simulink model "Untitled1"  (R2022a)
settings: Solver=VariableStepAuto  StartTime=0.0  StopTime=20  RelTol=1e-3
undefined symbols (not defined in the file or in its folder): X, Y, Z
libraries: sm_lib x10, nesl_utility x6
settings Model: SimulationMode=accelerator  Creator=alessiofranci  LastModifiedBy=alessiofranci

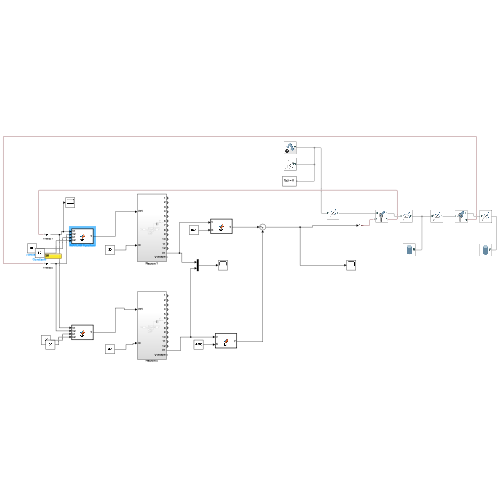
[thumbnail: Simulink's stored preview of the top-level diagram]
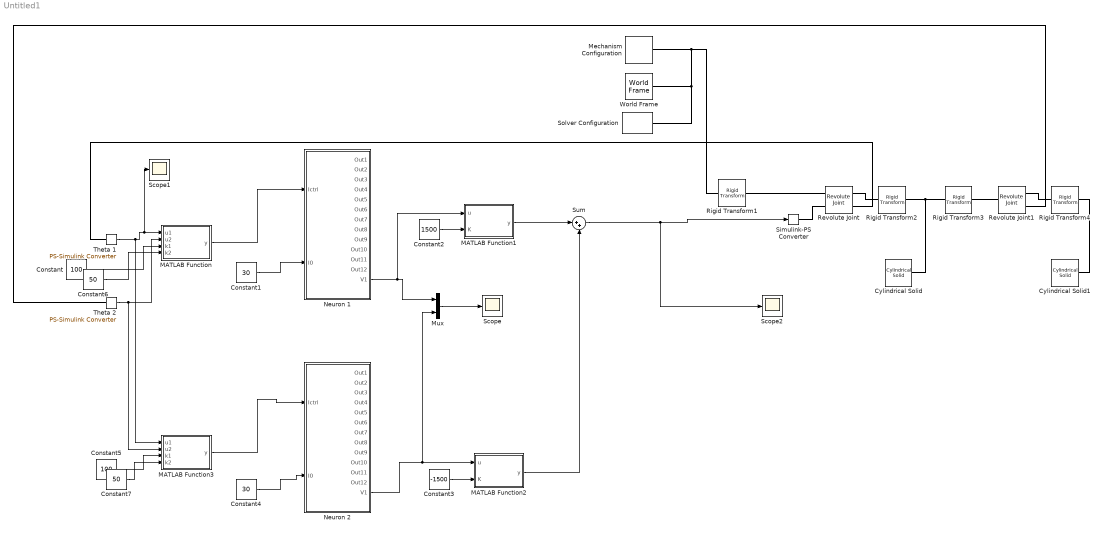
== system Untitled1 ==
  Constant : Constant  Value=100
  Constant1 : Constant  Value=30
  Constant2 : Constant  Value=1500
  Constant3 : Constant  Value=-1500
  Constant4 : Constant  Value=30
  Constant5 : Constant  Value=100
  Constant6 : Constant  Value=50
  Constant7 : Constant  Value=50
  Cylindrical Solid : sm_lib/Body Elements/Cylindrical Solid  GraphicAmbientColor=[0.15 0.15 0.15 1.0]  BasedOnType=Density  CenterOfMass=[0 0 0]  CenterOfMassUnits=m  GraphicDiffuseColor=[0.5 0.5 0.5]  CylinderLength=0.5  CylinderLengthUnits=m  CylinderRadius=0.05  CylinderRadiusUnits=m  Density=1000  DensityUnits=kg/m^3  DoExposeReferenceFrame=on  GraphicEmissiveColor=[0.0 0.0 0.0 1.0]  ExportEntireGeometry=off  SerializedFrames=<Frames/>  MarkerShape=Sphere  MarkerSize=10  GraphicType=FromGeometry  InertiaType=CalculateFromGeometry  Mass=1  MassUnits=kg  MomentsOfInertia=[1 1 1]  MomentsOfInertiaUnits=kg*m^2  GraphicOpacity=1.0  ProductsOfInertia=[0 0 0]  ProductsOfInertiaUnits=kg*m^2  GraphicShininess=75  GraphicSpecularColor=[0.5 0.5 0.5 1.0]  GraphicVisPropType=SimpleVisualProperties
  Cylindrical Solid1 : sm_lib/Body Elements/Cylindrical Solid  GraphicAmbientColor=[0.15 0.15 0.15 1.0]  BasedOnType=Density  CenterOfMass=[0 0 0]  CenterOfMassUnits=m  GraphicDiffuseColor=[0.5 0.5 0.5]  CylinderLength=0.5  CylinderLengthUnits=m  CylinderRadius=0.05  CylinderRadiusUnits=m  Density=1000  DensityUnits=kg/m^3  DoExposeReferenceFrame=on  GraphicEmissiveColor=[0.0 0.0 0.0 1.0]  ExportEntireGeometry=off  SerializedFrames=<Frames/>  MarkerShape=Sphere  MarkerSize=10  GraphicType=FromGeometry  InertiaType=CalculateFromGeometry  Mass=1  MassUnits=kg  MomentsOfInertia=[1 1 1]  MomentsOfInertiaUnits=kg*m^2  GraphicOpacity=1.0  ProductsOfInertia=[0 0 0]  ProductsOfInertiaUnits=kg*m^2  GraphicShininess=75  GraphicSpecularColor=[0.5 0.5 0.5 1.0]  GraphicVisPropType=SimpleVisualProperties
  MATLAB Function : MATLAB Function  TreatAsAtomicUnit=on
  MATLAB Function1 : MATLAB Function  TreatAsAtomicUnit=on
  MATLAB Function2 : MATLAB Function  TreatAsAtomicUnit=on
  MATLAB Function3 : MATLAB Function  TreatAsAtomicUnit=on
  Mechanism Configuration : sm_lib/Utilities/Mechanism Configuration  UniformGravity=Constant  GravityVector=[0 0 -9.80665]  GravityUnits=m/s^2  LinearizationDelta=0.001  JointModeTransitionNonlinearIterations=2
  Mux : Mux  Inputs=2
  Neuron 1 : Subsystem
  Neuron 2 : Subsystem
  Revolute Joint : sm_lib/Joints/Revolute Joint  JointMode=Normal  SenseConstraintForce=off  SenseConstraintForceX=off  SenseConstraintForceY=off  SenseConstraintForceZ=off  SenseConstraintTorque=off  SenseConstraintTorqueX=off  SenseConstraintTorqueY=off  SenseConstraintTorqueZ=off  SenseTotalForce=off  SenseTotalForceX=off  SenseTotalForceY=off  SenseTotalForceZ=off  SenseTotalTorque=off  SenseTotalTorqueX=off  SenseTotalTorqueY=off  SenseTotalTorqueZ=off  CompositeWrenchDir=FollowerOnBase  CompositeWrenchFrame=BaseFrame  EquilibriumPosition=0  EquilibriumPositionUnits=deg  SpringStiffness=0.0  SpringStiffnessUnits=N*m/deg  DampingCoefficient=0.0  DampingCoefficientUnits=N*m/(deg/s)  TorqueActuationMode=InputTorque  MotionActuationMode=ComputedMotion  SensePosition=on  SenseVelocity=off  SenseAcceleration=off  SenseTorqueForce=off  SenseLowerLimitTorqueForce=off  SenseUpperLimitTorqueForce=off  LowerLimitSpecify=off  LowerLimitBound=-90  LowerLimitBoundUnits=deg  LowerLimitStiffness=1e4  LowerLimitStiffnessUnits=N*m/deg  LowerLimitDamping=10  LowerLimitDampingUnits=N*m/(deg/s)  LowerLimitTransitionRegionWidth=0.1  LowerLimitTransitionRegionWidthUnits=deg  UpperLimitSpecify=off  UpperLimitBound=90  UpperLimitBoundUnits=deg  UpperLimitStiffness=1e4  UpperLimitStiffnessUnits=N*m/deg  UpperLimitDamping=10  UpperLimitDampingUnits=N*m/(deg/s)  UpperLimitTransitionRegionWidth=0.1  UpperLimitTransitionRegionWidthUnits=deg  PositionTargetSpecify=on  PositionTargetPriority=High  PositionTargetValue=20  PositionTargetValueUnits=deg  VelocityTargetSpecify=off  VelocityTargetPriority=High  VelocityTargetValue=0  VelocityTargetValueUnits=deg/s
  Revolute Joint1 : sm_lib/Joints/Revolute Joint  JointMode=Normal  SenseConstraintForce=off  SenseConstraintForceX=off  SenseConstraintForceY=off  SenseConstraintForceZ=off  SenseConstraintTorque=off  SenseConstraintTorqueX=off  SenseConstraintTorqueY=off  SenseConstraintTorqueZ=off  SenseTotalForce=off  SenseTotalForceX=off  SenseTotalForceY=off  SenseTotalForceZ=off  SenseTotalTorque=off  SenseTotalTorqueX=off  SenseTotalTorqueY=off  SenseTotalTorqueZ=off  CompositeWrenchDir=FollowerOnBase  CompositeWrenchFrame=BaseFrame  EquilibriumPosition=0  EquilibriumPositionUnits=deg  SpringStiffness=0.0  SpringStiffnessUnits=N*m/deg  DampingCoefficient=0.0  DampingCoefficientUnits=N*m/(deg/s)  TorqueActuationMode=NoTorque  MotionActuationMode=ComputedMotion  SensePosition=on  SenseVelocity=off  SenseAcceleration=off  SenseTorqueForce=off  SenseLowerLimitTorqueForce=off  SenseUpperLimitTorqueForce=off  LowerLimitSpecify=off  LowerLimitBound=-90  LowerLimitBoundUnits=deg  LowerLimitStiffness=1e4  LowerLimitStiffnessUnits=N*m/deg  LowerLimitDamping=10  LowerLimitDampingUnits=N*m/(deg/s)  LowerLimitTransitionRegionWidth=0.1  LowerLimitTransitionRegionWidthUnits=deg  UpperLimitSpecify=off  UpperLimitBound=90  UpperLimitBoundUnits=deg  UpperLimitStiffness=1e4  UpperLimitStiffnessUnits=N*m/deg  UpperLimitDamping=10  UpperLimitDampingUnits=N*m/(deg/s)  UpperLimitTransitionRegionWidth=0.1  UpperLimitTransitionRegionWidthUnits=deg  PositionTargetSpecify=on  PositionTargetPriority=High  PositionTargetValue=-20  PositionTargetValueUnits=deg  VelocityTargetSpecify=off  VelocityTargetPriority=High  VelocityTargetValue=0  VelocityTargetValueUnits=deg/s
  Rigid Transform1 : sm_lib/Frames and Transforms/Rigid Transform  TranslationMethod=None  TranslationStandardOffset=0.25  TranslationLengthUnit=m  TranslationStandardAxis=+X  TranslationCartesianOffset=[0 0 0]  TranslationROffset=0  TranslationROffsetUnits=m  TranslationZOffset=0  TranslationZOffsetUnits=m  TranslationThetaOffset=0  TranslationThetaOffsetUnits=deg  RotationMethod=RotationSequence  RotationAngleUnits=deg  RotationStandardAxis=+Y  RotationAngle=90  RotationArbitraryAxis=[0 0 1]  FollAlignAxisA=+X  BaseAlignAxisA=+Y  FollAlignAxisB=+Y  BaseAlignAxisB=+Z  RotationSequenceAxes=FollowerAxes  RotationSequence=XYX  RotationSequenceAngles=[0 90 90]  RotationSequenceAnglesUnits=deg  RotationMatrix=[1 0 0; 0 1 0; 0 0 1]
  Rigid Transform2 : sm_lib/Frames and Transforms/Rigid Transform  TranslationMethod=StandardAxis  TranslationStandardOffset=.25  TranslationLengthUnit=m  TranslationStandardAxis=+X  TranslationCartesianOffset=[0 0 0]  TranslationROffset=0  TranslationROffsetUnits=m  TranslationZOffset=0  TranslationZOffsetUnits=m  TranslationThetaOffset=0  TranslationThetaOffsetUnits=deg  RotationMethod=RotationSequence  RotationAngleUnits=deg  RotationStandardAxis=+Z  RotationAngle=90  RotationArbitraryAxis=[0 0 1]  FollAlignAxisA=+X  BaseAlignAxisA=+Y  FollAlignAxisB=+Y  BaseAlignAxisB=+Z  RotationSequenceAxes=FollowerAxes  RotationSequence=XYX  RotationSequenceAngles=[0 90 0]  RotationSequenceAnglesUnits=deg  RotationMatrix=[1 0 0; 0 1 0; 0 0 1]
  Rigid Transform3 : sm_lib/Frames and Transforms/Rigid Transform  TranslationMethod=StandardAxis  TranslationStandardOffset=.25  TranslationLengthUnit=m  TranslationStandardAxis=+Z  TranslationCartesianOffset=[0 0 0]  TranslationROffset=0  TranslationROffsetUnits=m  TranslationZOffset=0  TranslationZOffsetUnits=m  TranslationThetaOffset=0  TranslationThetaOffsetUnits=deg  RotationMethod=RotationSequence  RotationAngleUnits=deg  RotationStandardAxis=+Z  RotationAngle=90  RotationArbitraryAxis=[0 0 1]  FollAlignAxisA=+X  BaseAlignAxisA=+Y  FollAlignAxisB=+Y  BaseAlignAxisB=+Z  RotationSequenceAxes=FollowerAxes  RotationSequence=XYX  RotationSequenceAngles=[0 -90 0]  RotationSequenceAnglesUnits=deg  RotationMatrix=[1 0 0; 0 1 0; 0 0 1]
  Rigid Transform4 : sm_lib/Frames and Transforms/Rigid Transform  TranslationMethod=StandardAxis  TranslationStandardOffset=.25  TranslationLengthUnit=m  TranslationStandardAxis=+X  TranslationCartesianOffset=[0 0 0]  TranslationROffset=0  TranslationROffsetUnits=m  TranslationZOffset=0  TranslationZOffsetUnits=m  TranslationThetaOffset=0  TranslationThetaOffsetUnits=deg  RotationMethod=RotationSequence  RotationAngleUnits=deg  RotationStandardAxis=+Z  RotationAngle=90  RotationArbitraryAxis=[0 0 1]  FollAlignAxisA=+X  BaseAlignAxisA=+Y  FollAlignAxisB=+Y  BaseAlignAxisB=+Z  RotationSequenceAxes=FollowerAxes  RotationSequence=XYZ  RotationSequenceAngles=[0 90 0]  RotationSequenceAnglesUnits=deg  RotationMatrix=[1 0 0; 0 1 0; 0 0 1]
  Scope : Scope
  Scope1 : Scope
  Scope2 : Scope
  Simulink-PS Converter : nesl_utility/Simulink-PS Converter  PhysicalDomain=network_engine_domain  SubClassName=ps_input  LeftPortType=input  RightPortType=output  PseudoPeriodic=off  Frequencies=[]  NoiseDistribution=none  NoiseParameters=[]  Unit=1  AffineConversion=off  FilteringAndDerivatives=provide  SimscapeFilterOrder=1  InputFilterTimeConstant=0.001  UdotUserProvided=0
      settings: SourceProductBaseCode=SS,PW,VE
  Solver Configuration : nesl_utility/Solver Configuration  PhysicalDomain=network_engine_domain  SubClassName=solver  LeftPortType=input  RightPortType=generic  Tones=[]  Harmonics=[]  SimulateNoise=off  Profile=off  UseLocalSampling=off  EnableSwitchedLinearOptims=on  FrequencyDomain=off  UseCCode=off  RelTol=0.001  AbsTol=1e-06  MinStep=1e-09  ToWorkspace=off  RevertToSquareIcSolve=off  NumHomotopyIterations=100  PhasorMode=off  PhasorModeNumHarmonics=1  IndexReductionMethod=DerivativeReplacement  DoDC=off  ResidualTolerance=1e-09  UseLocalSolver=off  LocalSolverChoice=NE_BACKWARD_EULER_ADVANCER  LocalSolverSampleTime=0.001  DoFixedCost=off  MaxNonlinIter=3  MaxModeIter=2  ComputeImpulses=off  ImpulseIterations=2  LinearAlgebra=auto  LinearAlgebraNumThread=0  EquationFormulation=NE_TIME_EF  DelaysMemoryBudget=1024  AutomaticFiltering=on  FilteringTimeConstant=0.001  PartitionStorageMethod=AS_NEEDED  PartitionMemoryBudget=1024  PartitionMethod=ROBUST
      settings: SourceProductBaseCode=SS,PW,VE
  Sum : Sum  Inputs=|++
  Theta 1 : nesl_utility/PS-Simulink Converter  PhysicalDomain=network_engine_domain  SubClassName=ps_output  LeftPortType=input  RightPortType=output  PseudoPeriodic=off  Frequencies=[]  VectorFormat=inherit  Unit=inherit  AffineConversion=off
      settings: SourceProductBaseCode=SS,PW,VE
  Theta 2 : nesl_utility/PS-Simulink Converter  PhysicalDomain=network_engine_domain  SubClassName=ps_output  LeftPortType=input  RightPortType=output  PseudoPeriodic=off  Frequencies=[]  VectorFormat=inherit  Unit=inherit  AffineConversion=off
      settings: SourceProductBaseCode=SS,PW,VE
  World Frame : sm_lib/Frames and Transforms/World Frame
  wires:
  Mux/1 -> Scope/1
  Neuron 1/13(V1) -> MATLAB Function1/1(u), Mux/1
  Theta 1/1 -> MATLAB Function3/1(u1), Scope1/1, MATLAB Function/1(u1)
  MATLAB Function/1(y) -> Neuron 1/1(Ictrl)
  Constant1/1 -> Neuron 1/2(I0)
  Constant2/1 -> MATLAB Function1/2(K)
  MATLAB Function1/1(y) -> Sum/1
  Sum/1 -> Scope2/1, Simulink-PS Converter/1
  Neuron 2/13(V1) -> Mux/2, MATLAB Function2/1(u)
  MATLAB Function2/1(y) -> Sum/2
  Constant3/1 -> MATLAB Function2/2(K)
  Constant4/1 -> Neuron 2/2(I0)
  MATLAB Function3/1(y) -> Neuron 2/1(Ictrl)
  Theta 2/1 -> MATLAB Function/2(u2), MATLAB Function3/2(u2)
  Constant6/1 -> MATLAB Function/4(k2)
  Constant5/1 -> MATLAB Function3/3(k1)
  Constant7/1 -> MATLAB Function3/4(k2)
  Constant/1 -> MATLAB Function/3(k1)
  connections:
  Cylindrical Solid/RConn1 -- Rigid Transform2/RConn1 -- Rigid Transform3/LConn1
  Mechanism Configuration/RConn1 -- Solver Configuration/RConn1 -- World Frame/RConn1 -- Rigid Transform1/LConn1
  Revolute Joint1/RConn1 -- Rigid Transform4/LConn1
  Rigid Transform2/LConn1 -- Revolute Joint/RConn1
  Revolute Joint1/LConn1 -- Rigid Transform3/RConn1
  Rigid Transform4/RConn1 -- Cylindrical Solid1/RConn1
  Rigid Transform1/RConn1 -- Revolute Joint/LConn1
  Simulink-PS Converter/RConn1 -- Revolute Joint/LConn2
  Revolute Joint/RConn2 -- Theta 1/LConn1
  Revolute Joint1/RConn2 -- Theta 2/LConn1

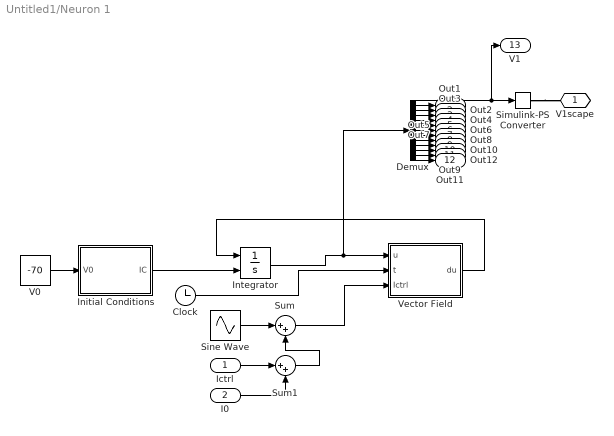
== system Untitled1/Neuron 1 ==
  Ictrl : Inport
  I0 : Inport  Port=2
  Clock : Clock
  Demux : Demux  Outputs=13
  Initial Conditions : MATLAB Function  TreatAsAtomicUnit=on
  Integrator : Integrator  InitialConditionSource=external  InitialCondition=[-70,]
  Simulink-PS Converter : nesl_utility/Simulink-PS Converter  PhysicalDomain=network_engine_domain  SubClassName=ps_input  LeftPortType=input  RightPortType=output  PseudoPeriodic=off  Frequencies=[]  NoiseDistribution=none  NoiseParameters=[]  Unit=1  AffineConversion=off  FilteringAndDerivatives=provide  SimscapeFilterOrder=1  InputFilterTimeConstant=0.001  UdotUserProvided=0
      settings: SourceProductBaseCode=SS,PW,VE
  Sine Wave : Sin  Amplitude=0  Frequency=0.002  SampleTime=0
  Sum : Sum  Inputs=|++
  Sum1 : Sum  Inputs=|++
  V0 : Constant  Value=-70
  Vector Field : MATLAB Function  TreatAsAtomicUnit=on
  V1scape : PMIOPort  Side=Right
  Out1 : Outport
  Out2 : Outport  Port=2
  Out3 : Outport  Port=3
  Out4 : Outport  Port=4
  Out5 : Outport  Port=5
  Out6 : Outport  Port=6
  Out7 : Outport  Port=7
  Out8 : Outport  Port=8
  Out9 : Outport  Port=9
  Out10 : Outport  Port=10
  Out11 : Outport  Port=11
  Out12 : Outport  Port=12
  V1 : Outport  Port=13
  wires:
  Demux/13 -> Out12/1
  Demux/2 -> Out1/1
  Demux/3 -> Out2/1
  Demux/5 -> Out4/1
  Demux/9 -> Out8/1
  Demux/11 -> Out10/1
  Demux/8 -> Out7/1
  V0/1 -> Initial Conditions/1(V0)
  Demux/1 -> V1/1, Simulink-PS Converter/1
  Sum/1 -> Vector Field/3(Ictrl)
  Demux/10 -> Out9/1
  Clock/1 -> Vector Field/2(t)
  Demux/6 -> Out5/1
  Demux/4 -> Out3/1
  Initial Conditions/1(IC) -> Integrator/2
  Integrator/1 -> Demux/1, Vector Field/1(u)
  Demux/7 -> Out6/1
  Vector Field/1(du) -> Integrator/1
  Demux/12 -> Out11/1
  Sine Wave/1 -> Sum/1
  Sum1/1 -> Sum/2
  Ictrl/1 -> Sum1/1
  I0/1 -> Sum1/2
  connections:
  Simulink-PS Converter/RConn1 -- V1scape/RConn1

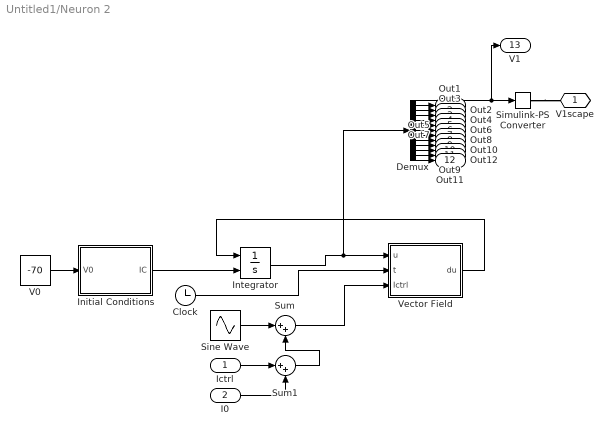
== system Untitled1/Neuron 2 ==
  Ictrl : Inport
  I0 : Inport  Port=2
  Clock : Clock
  Demux : Demux  Outputs=13
  Initial Conditions : MATLAB Function  TreatAsAtomicUnit=on
  Integrator : Integrator  InitialConditionSource=external  InitialCondition=[-70,]
  Simulink-PS Converter : nesl_utility/Simulink-PS Converter  PhysicalDomain=network_engine_domain  SubClassName=ps_input  LeftPortType=input  RightPortType=output  PseudoPeriodic=off  Frequencies=[]  NoiseDistribution=none  NoiseParameters=[]  Unit=1  AffineConversion=off  FilteringAndDerivatives=provide  SimscapeFilterOrder=1  InputFilterTimeConstant=0.001  UdotUserProvided=0
      settings: SourceProductBaseCode=SS,PW,VE
  Sine Wave : Sin  Amplitude=0  Frequency=0.002  SampleTime=0
  Sum : Sum  Inputs=|++
  Sum1 : Sum  Inputs=|++
  V0 : Constant  Value=-70
  Vector Field : MATLAB Function  TreatAsAtomicUnit=on
  V1scape : PMIOPort  Side=Right
  Out1 : Outport
  Out2 : Outport  Port=2
  Out3 : Outport  Port=3
  Out4 : Outport  Port=4
  Out5 : Outport  Port=5
  Out6 : Outport  Port=6
  Out7 : Outport  Port=7
  Out8 : Outport  Port=8
  Out9 : Outport  Port=9
  Out10 : Outport  Port=10
  Out11 : Outport  Port=11
  Out12 : Outport  Port=12
  V1 : Outport  Port=13
  wires:
  Demux/13 -> Out12/1
  Demux/2 -> Out1/1
  Demux/3 -> Out2/1
  Demux/5 -> Out4/1
  Demux/9 -> Out8/1
  Demux/11 -> Out10/1
  Demux/8 -> Out7/1
  V0/1 -> Initial Conditions/1(V0)
  Demux/1 -> V1/1, Simulink-PS Converter/1
  Sum/1 -> Vector Field/3(Ictrl)
  Demux/10 -> Out9/1
  Clock/1 -> Vector Field/2(t)
  Demux/6 -> Out5/1
  Demux/4 -> Out3/1
  Initial Conditions/1(IC) -> Integrator/2
  Integrator/1 -> Demux/1, Vector Field/1(u)
  Demux/7 -> Out6/1
  Vector Field/1(du) -> Integrator/1
  Demux/12 -> Out11/1
  Sine Wave/1 -> Sum/1
  Sum1/1 -> Sum/2
  Ictrl/1 -> Sum1/1
  I0/1 -> Sum1/2
  connections:
  Simulink-PS Converter/RConn1 -- V1scape/RConn1

== matlab function Untitled1/Neuron 1/Initial Conditions ==
  data: V0 input; IC output
function IC = fcn(V0)

VCa = 120.;
aa=0.1;
bb=0.1;
gCaL=0.;
gCaT=0.;

mNa0=mNainf(V0);
hNa0=hNainf(V0);
mKd0=mKdinf(V0);
mAf0=mAfinf(V0); 
hAf0=hAfinf(V0); 
mAs0=mAsinf(V0); 
hAs0=hAsinf(V0); 
mCaL0=mCaLinf(V0); 
mCaT0=mCaTinf(V0); 
hCaT0=hCaTinf(V0); 
mH0=mHinf(V0);
Ca0=(-aa*gCaL*mCaL0*(V0-VCa))+(-bb*gCaT*mCaT0*hCaT0*(V0-VCa));

IC = [V0; mNa0; hNa0; mKd0; mAf0; hAf0; mAs0; hAs0; mCaL0; mCaT0; hCaT0; mH0; Ca0];
end

% Model gating functions
% All activation and inactivation curves are defined by the Boltzman function

function out = Xinf(V,A,B)
    out = 1.0 ./ (1+exp((V+A)/B));
end

% All timeconstant curves are defined by the shifted Boltzman function

function out = tauX(V,A,B,D,E)
    out = A-B./(1+exp((V+D)/E));
end

% Sodium current

function out = mNainf(V)
    out = Xinf(V,25.0,-5.0);
end


function out = hNainf(V)
    out = Xinf(V,40.,10.);
end

% Potassium currents

function out = mKdinf(V)
    out = Xinf(V,15.,-10.);
end


function out = mAfinf(V)
    out = Xinf(V,80,-10.);
end

function out = hAfinf(V)
    out = Xinf(V,60,5.);
end


function out = mAsinf(V)
    out = Xinf(V,60,-10.);
end

function out = hAsinf(V)
    out = Xinf(V,20,5.);
end


% # Calcium currents

function out = mCaLinf(V)
    out = Xinf(V,45.,-5.);
end

function out = mCaTinf(V)
    out = Xinf(V,60,-5.);
end


function out = hCaTinf(V)
    out = Xinf(V,85,10.);
end


% # Cation current (H-current)

function out = mHinf(V)
    out = Xinf(V,85,10.);
end

== matlab function Untitled1/Neuron 1/Vector Field ==
  data: u input; du output; t input; Ictrl input
function du = fcn(u,t,Ictrl)

VNa = 40.; 
VK = -90.; 
VCa = 120.;
VH= -40.;
Vl = -50.;
C=0.1;
aa=0.1;
bb=0.1;
 
gl=0.3;
gNa=100.;
gKd=65.;
gAf=15.0; 
gAs=0.; 
gKCa=0.;
gCaL=0.;
gCaT=0.;
gH=0.;

Iapp=200.0;%217.8;  Close to reobase, which is around 228.

I1=0.0;%10.; 
ti1=500;
tf1=2500; 

I2=0.0;%10.5; 
ti2=3500; 
tf2=5500; 

% Variables
V=u(1); % Membrane potential
mNa=u(2); % Sodium current activation
hNa=u(3); % Sodium current inactivation
mKd=u(4); % Delayed-rectifier potassium current activation
mAf=u(5); % Fast A-type potassium current activation
hAf=u(6); % Fast A-type potassium current inactivation
mAs=u(7); % Slow A-type potassium current activation
hAs=u(8); % Slow A-type potassium current inactivation
mCaL=u(9); % L-type calcium current activation
mCaT=u(10); % T-type calcium current activation
hCaT=u(11); % T-type calcium current inactivation
mH=u(12); % H current activation
Ca=u(13); % Intracellular calcium concentration

du = zeros(13,1);

du(1) = 1000*(1/C) * (-gNa*mNa*hNa*(V-VNa) + ...
-gKd*mKd*(V-VK) -gAf*mAf*hAf*(V-VK) -gAs*mAs*hAs*(V-VK) + ...
-gKCa*mKCainf(Ca)*(V-VK) + ...
-gCaL*mCaL*(V-VCa) + ...
-gCaT*mCaT*hCaT*(V-VCa) + ...
-gH*mH*(V-VH) + ...
-gl*(V-Vl) + ...
+Iapp + I1*pulse(t,ti1,tf1) + I2*pulse(t,ti2,tf2)+Ictrl);
du(2) = 1000*(1/tau_mNa(V)) * (mNainf(V) - mNa);
du(3) = 1000*(1/tau_hNa(V)) * (hNainf(V) - hNa);
du(4) = 1000*(1/tau_mKd(V)) * (mKdinf(V) - mKd);
du(5) = 1000*(1/tau_mAf(V)) * (mAfinf(V) - mAf);
du(6) = 1000*(1/tau_hAf(V)) * (hAfinf(V) - hAf);
du(7) = 1000*(1/tau_mAs(V)) * (mAsinf(V) - mAs);
du(8) = 1000*(1/tau_hAs(V)) * (hAsinf(V) - hAs);
du(9) = 1000*(1/tau_mCaL(V)) * (mCaLinf(V) - mCaL);
du(10) = 1000*(1/tau_mCaT(V)) * (mCaTinf(V) - mCaT);
du(11) = 1000*(1/tau_hCaT(V)) * (hCaTinf(V) - hCaT);
du(12) = 1000*(1/tau_mH(V)) * (mHinf(V) - mH);
du(13) = 1000*(1/tau_Ca()) * ((-aa*gCaL*mCaL*(V-VCa))+(-bb*gCaT*mCaT*hCaT*(V-VCa)) - Ca);
end

function out = heaviside(t)
    out = (1+sign(t))/2;
end

function out = pulse(t,ti,tf)
    out = heaviside(t-ti)-heaviside(t-tf);
end

% Model gating functions
% All activation and inactivation curves are defined by the Boltzman function

function out = Xinf(V,A,B)
    out = 1.0 ./ (1+exp((V+A)/B));
end

% All timeconstant curves are defined by the shifted Boltzman function

function out = tauX(V,A,B,D,E)
    out = A-B./(1+exp((V+D)/E));
end

% Sodium current

function out = mNainf(V)
    out = Xinf(V,25.0,-5.0);
end

function out = tau_mNa(V)
    out = tauX(V,0.75,0.5,100.,-20.);
end

function out = hNainf(V)
    out = Xinf(V,40.,10.);
end

function out = tau_hNa(V)
    out = tauX(V,4.0,3.5,50.,-20.);
end

% Potassium currents

function out = mKdinf(V)
    out = Xinf(V,15.,-10.);
end

function out = tau_mKd(V)
    out = tauX(V,5.0,4.5,30.,-20.);
end

function out = mAfinf(V)
    out = Xinf(V,80,-10.);
end

function out = tau_mAf(V)
    out = tauX(V,0.75,0.5,100.,-20.);
end

function out = hAfinf(V)
    out = Xinf(V,60,5.);
end

function out = tau_hAf(V)
    out = 10*tauX(V,0.75,0.5,100.,-20.);
end

function out = mAsinf(V)
    out = Xinf(V,60,-10.);
end

function out = tau_mAs(V)
    out = 10*tauX(V,0.75,0.5,100.,-20.);
end

function out = hAsinf(V)
    out = Xinf(V,20,5.);
end

function out = tau_hAs(V)
    out = 100*tauX(V,0.75,0.5,100.,-20.);
end

function out = mKCainf(Ca)
    out = Xinf(Ca,-30.0,-10.);
end

% # Calcium currents

function out = mCaLinf(V)
    out = Xinf(V,45.,-5.);
end

function out = tau_mCaL(V)
    out = tauX(V,6.0,5.5,30.,-20.);
end

function out = mCaTinf(V)
    out = Xinf(V,60,-5.);
end

function out = tau_mCaT(V)
    out = tauX(V,6.0,5.5,30.,-20.);
end

function out = hCaTinf(V)
    out = Xinf(V,85,10.);
end

function out = tau_hCaT(V)
    out = 100*tauX(V,6.0,5.5,30.,-20.);
end

% # Cation current (H-current)

function out = mHinf(V)
    out = Xinf(V,85,10.);
end

function out = tau_mH(V)
    out = 50*tauX(V,6.0,5.5,30.,-20.);
end

function out = tau_Ca()

    out = 500.0;
end

== matlab function Untitled1/MATLAB Function1 ==
  data: u input; y output; K input
function y = fcn(u,K)

y = K/(1+exp(-(u+20)));

== matlab function Untitled1/Neuron 2/Initial Conditions ==
  data: V0 input; IC output
function IC = fcn(V0)

VCa = 120.;
aa=0.1;
bb=0.1;
gCaL=0.;
gCaT=0.;

mNa0=mNainf(V0);
hNa0=hNainf(V0);
mKd0=mKdinf(V0);
mAf0=mAfinf(V0); 
hAf0=hAfinf(V0); 
mAs0=mAsinf(V0); 
hAs0=hAsinf(V0); 
mCaL0=mCaLinf(V0); 
mCaT0=mCaTinf(V0); 
hCaT0=hCaTinf(V0); 
mH0=mHinf(V0);
Ca0=(-aa*gCaL*mCaL0*(V0-VCa))+(-bb*gCaT*mCaT0*hCaT0*(V0-VCa));

IC = [V0; mNa0; hNa0; mKd0; mAf0; hAf0; mAs0; hAs0; mCaL0; mCaT0; hCaT0; mH0; Ca0];
end

% Model gating functions
% All activation and inactivation curves are defined by the Boltzman function

function out = Xinf(V,A,B)
    out = 1.0 ./ (1+exp((V+A)/B));
end

% All timeconstant curves are defined by the shifted Boltzman function

function out = tauX(V,A,B,D,E)
    out = A-B./(1+exp((V+D)/E));
end

% Sodium current

function out = mNainf(V)
    out = Xinf(V,25.0,-5.0);
end


function out = hNainf(V)
    out = Xinf(V,40.,10.);
end

% Potassium currents

function out = mKdinf(V)
    out = Xinf(V,15.,-10.);
end


function out = mAfinf(V)
    out = Xinf(V,80,-10.);
end

function out = hAfinf(V)
    out = Xinf(V,60,5.);
end


function out = mAsinf(V)
    out = Xinf(V,60,-10.);
end

function out = hAsinf(V)
    out = Xinf(V,20,5.);
end


% # Calcium currents

function out = mCaLinf(V)
    out = Xinf(V,45.,-5.);
end

function out = mCaTinf(V)
    out = Xinf(V,60,-5.);
end


function out = hCaTinf(V)
    out = Xinf(V,85,10.);
end


% # Cation current (H-current)

function out = mHinf(V)
    out = Xinf(V,85,10.);
end

== matlab function Untitled1/MATLAB Function ==
  data: u1 input; y output; u2 input; k1 input; k2 input
function y = fcn(u1,u2,k1,k2)

y = -k1*sin((u1-pi-0.1))+k2*sin(u2);

== matlab function Untitled1/Neuron 2/Vector Field ==
  data: u input; du output; t input; Ictrl input
function du = fcn(u,t,Ictrl)

VNa = 40.; 
VK = -90.; 
VCa = 120.;
VH= -40.;
Vl = -50.;
C=0.1;
aa=0.1;
bb=0.1;
 
gl=0.3;
gNa=100.;
gKd=65.;
gAf=15.0; 
gAs=0.; 
gKCa=0.;
gCaL=0.;
gCaT=0.;
gH=0.;

Iapp=200.0;%217.8;  Close to reobase, which is around 228.

I1=0.0;%10.; 
ti1=500;
tf1=2500; 

I2=0.0;%10.5; 
ti2=3500; 
tf2=5500; 

% Variables
V=u(1); % Membrane potential
mNa=u(2); % Sodium current activation
hNa=u(3); % Sodium current inactivation
mKd=u(4); % Delayed-rectifier potassium current activation
mAf=u(5); % Fast A-type potassium current activation
hAf=u(6); % Fast A-type potassium current inactivation
mAs=u(7); % Slow A-type potassium current activation
hAs=u(8); % Slow A-type potassium current inactivation
mCaL=u(9); % L-type calcium current activation
mCaT=u(10); % T-type calcium current activation
hCaT=u(11); % T-type calcium current inactivation
mH=u(12); % H current activation
Ca=u(13); % Intracellular calcium concentration

du = zeros(13,1);

du(1) = 1000*(1/C) * (-gNa*mNa*hNa*(V-VNa) + ...
-gKd*mKd*(V-VK) -gAf*mAf*hAf*(V-VK) -gAs*mAs*hAs*(V-VK) + ...
-gKCa*mKCainf(Ca)*(V-VK) + ...
-gCaL*mCaL*(V-VCa) + ...
-gCaT*mCaT*hCaT*(V-VCa) + ...
-gH*mH*(V-VH) + ...
-gl*(V-Vl) + ...
+Iapp + I1*pulse(t,ti1,tf1) + I2*pulse(t,ti2,tf2)+Ictrl);
du(2) = 1000*(1/tau_mNa(V)) * (mNainf(V) - mNa);
du(3) = 1000*(1/tau_hNa(V)) * (hNainf(V) - hNa);
du(4) = 1000*(1/tau_mKd(V)) * (mKdinf(V) - mKd);
du(5) = 1000*(1/tau_mAf(V)) * (mAfinf(V) - mAf);
du(6) = 1000*(1/tau_hAf(V)) * (hAfinf(V) - hAf);
du(7) = 1000*(1/tau_mAs(V)) * (mAsinf(V) - mAs);
du(8) = 1000*(1/tau_hAs(V)) * (hAsinf(V) - hAs);
du(9) = 1000*(1/tau_mCaL(V)) * (mCaLinf(V) - mCaL);
du(10) = 1000*(1/tau_mCaT(V)) * (mCaTinf(V) - mCaT);
du(11) = 1000*(1/tau_hCaT(V)) * (hCaTinf(V) - hCaT);
du(12) = 1000*(1/tau_mH(V)) * (mHinf(V) - mH);
du(13) = 1000*(1/tau_Ca()) * ((-aa*gCaL*mCaL*(V-VCa))+(-bb*gCaT*mCaT*hCaT*(V-VCa)) - Ca);
end

function out = heaviside(t)
    out = (1+sign(t))/2;
end

function out = pulse(t,ti,tf)
    out = heaviside(t-ti)-heaviside(t-tf);
end

% Model gating functions
% All activation and inactivation curves are defined by the Boltzman function

function out = Xinf(V,A,B)
    out = 1.0 ./ (1+exp((V+A)/B));
end

% All timeconstant curves are defined by the shifted Boltzman function

function out = tauX(V,A,B,D,E)
    out = A-B./(1+exp((V+D)/E));
end

% Sodium current

function out = mNainf(V)
    out = Xinf(V,25.0,-5.0);
end

function out = tau_mNa(V)
    out = tauX(V,0.75,0.5,100.,-20.);
end

function out = hNainf(V)
    out = Xinf(V,40.,10.);
end

function out = tau_hNa(V)
    out = tauX(V,4.0,3.5,50.,-20.);
end

% Potassium currents

function out = mKdinf(V)
    out = Xinf(V,15.,-10.);
end

function out = tau_mKd(V)
    out = tauX(V,5.0,4.5,30.,-20.);
end

function out = mAfinf(V)
    out = Xinf(V,80,-10.);
end

function out = tau_mAf(V)
    out = tauX(V,0.75,0.5,100.,-20.);
end

function out = hAfinf(V)
    out = Xinf(V,60,5.);
end

function out = tau_hAf(V)
    out = 10*tauX(V,0.75,0.5,100.,-20.);
end

function out = mAsinf(V)
    out = Xinf(V,60,-10.);
end

function out = tau_mAs(V)
    out = 10*tauX(V,0.75,0.5,100.,-20.);
end

function out = hAsinf(V)
    out = Xinf(V,20,5.);
end

function out = tau_hAs(V)
    out = 100*tauX(V,0.75,0.5,100.,-20.);
end

function out = mKCainf(Ca)
    out = Xinf(Ca,-30.0,-10.);
end

% # Calcium currents

function out = mCaLinf(V)
    out = Xinf(V,45.,-5.);
end

function out = tau_mCaL(V)
    out = tauX(V,6.0,5.5,30.,-20.);
end

function out = mCaTinf(V)
    out = Xinf(V,60,-5.);
end

function out = tau_mCaT(V)
    out = tauX(V,6.0,5.5,30.,-20.);
end

function out = hCaTinf(V)
    out = Xinf(V,85,10.);
end

function out = tau_hCaT(V)
    out = 100*tauX(V,6.0,5.5,30.,-20.);
end

% # Cation current (H-current)

function out = mHinf(V)
    out = Xinf(V,85,10.);
end

function out = tau_mH(V)
    out = 50*tauX(V,6.0,5.5,30.,-20.);
end

function out = tau_Ca()

    out = 500.0;
end

== matlab function Untitled1/MATLAB Function2 ==
  data: u input; y output; K input
function y = fcn(u,K)

y = K/(1+exp(-(u+20)));

== matlab function Untitled1/MATLAB Function3 ==
  data: u1 input; y output; u2 input; k1 input; k2 input
function y = fcn(u1,u2,k1,k2)

y = k1*sin((u1-pi+0.1))-k2*sin(u2);
